simulink model "BusCreator_virtual"  (R2017b)
settings: Solver=FixedStepDiscrete  StartTime=0.0  StopTime=10.0  FixedStep=0.200000  RelTol=1e-3
settings Model: Creator=The MathWorks, Inc.  LastModifiedBy=hbourbou
settings OptimizationCC: LifeSpan=inf
settings DebuggingCC: SFExecutionAtInitializationDiag=none
settings HardwareCC: ProdBitPerSizeT=32  ProdBitPerPtrDiffT=32  ProdWordSize=32  ProdHWDeviceType=Specified
settings CodeAppCC: StateflowObjectComments=on
settings ConfigComp: CovMetricSettings=dswe

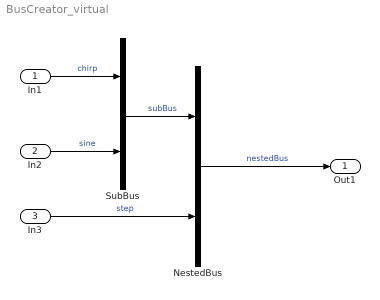
== system BusCreator_virtual ==
  In1 : Inport  PortDimensions=2
  In2 : Inport  Port=2  PortDimensions=3
  In3 : Inport  Port=3  PortDimensions=4
  NestedBus : BusCreator  Inputs=2
      settings: AttributesFormatString=NestedBus
  SubBus : BusCreator  Inputs=2
      settings: AttributesFormatString=SubBus
  Out1 : Outport
  wires:
  In1/1 -> SubBus/1  "chirp"
  SubBus/1 -> NestedBus/1  "subBus"
  In2/1 -> SubBus/2  "sine"
  In3/1 -> NestedBus/2  "step"
  NestedBus/1 -> Out1/1  "nestedBus"
